simulink model "TTS_4motor_simplify_PMSM_ver2"  (R2020b)
settings: Solver=VariableStepAuto  StartTime=0.0  StopTime=0.8  RelTol=1e-3
InitFcn:
  | C = 0.015 % 中间直流电路的电容
  | f = 50 %频率
  | Rn = 0.01 % 整流部分电阻
  | Ln = 0.0012; % 整流电路部分电感
  | Udcref = 800*sqrt(2)
  | Un = 350
  | 
  | noiseDense = 1e-4 % 速度传感器故障噪声
  | 
  | w = 2*pi*f
  | 
  | np=2;
  | Tloadmax  = 50 % 最大负载
  | Tloadstart = 0.35 % 负载添加时间
  | Tdiscrete = 2e-6 % 离散时间
  | t_precharge = 0.15 % 整流预充电
  | Tpwm = 5e-4 % 逆变 PWM 周期
  | Ts = 1e-4
  | sample_time = Tdiscrete; % scope 采样时间
  | 
  | %基础参数
  | Rs_ref=0.43
  | Lm_ref=0.0006931
  | J_ref=0.1
  | Rflux_ref = 0.175
  | 
  | 
  | %电机 1 参数
  | Rflux1=0.9618*Rflux_ref
  | Rs1=0.9874*Rs_ref
  | Lm1=0.9747*Lm_ref
  | J1=0.9645*J_ref
  | 
  | 
  | %电机 2 参数
  | Rflux2=1.0145*Rflux_ref
  | Rs2=0.9810*Rs_ref
  | Lm2=0.9963*Lm_ref
  | J2=1.0415*J_ref
  | 
  | 
  | %电机 3 参数
  | Rflux3=1.0317*Rflux_ref
  | Rs3=0.9948*Rs_ref
  | Lm3=0.9914*Lm_ref
  | J3=1.0269*J_ref
  | 
  | 
  | %电机 4 参数
  | Rflux4=1.0481*Rflux_ref
  | Rs4=0.9914*Rs_ref
  | Lm4=0.9938*Lm_ref
  | J4=0.9873*J_ref
  | 
  | 
  | 
  | % 故障设置参数
  | % 速度传感器
  | tE1w = 10.3
  | 
  | % 逆变器
  | 
  | 
  | m1_pB = 0
  | m1_pC = 0
  | m1_t_inverter = 0.4 % 逆变器故障发生的时间
  | 
  | m2_pA = 0
  | m2_pB = 0
  | m2_pC = 0
  | m2_t_inverter = 0.4 % 逆变器故障发生的时间
  | 
  | m3_pA = 0
  | m3_pB = 0
  | m3_pC = 0
  | m3_t_inverter = 0.4 % 逆变器故障发生的时间
  | 
  | m4_pA = 0
  | m4_pB = 0
  | m4_pC = 0
  | m4_t_inverter = 0.4 % 逆变器故障发生的时间
undefined symbols (not defined in the file): m1_pA
libraries: powerlib x23, simulink x11, pid_lib x1, eeSinusoidalMeasurementV2 x1
(part 1 of 2)
settings Model: SimulationMode=accelerator  OrderedModelArguments=off  Creator=messer  LastModifiedBy=messer
settings SolverCC: ZeroCrossAlgorithm=Adaptive
settings DebuggingCC: IgnoredZcDiagnostic=none

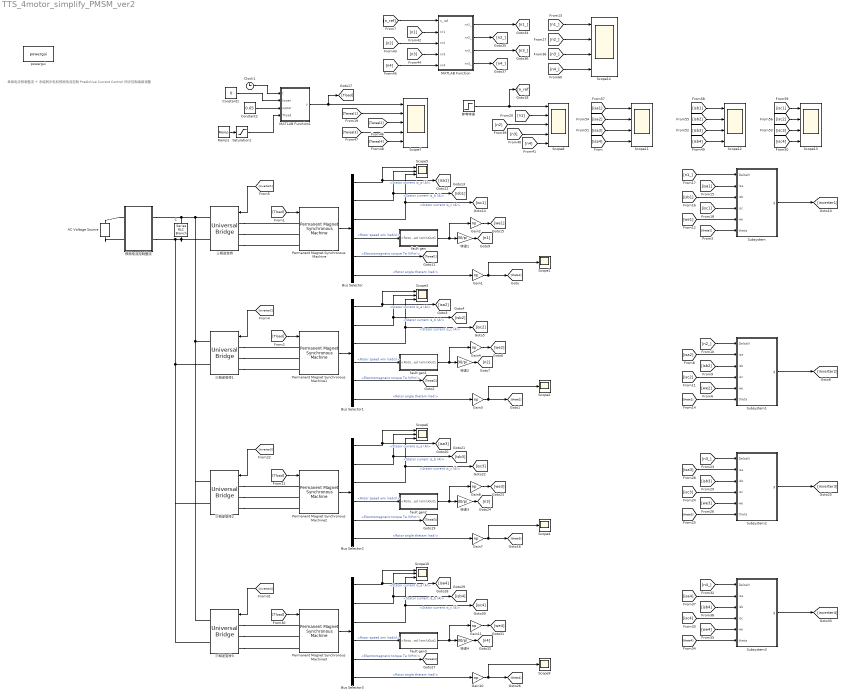
== system TTS_4motor_simplify_PMSM_ver2 ==
  note: 单相电流预测整流 + 永磁同步电机预测电流控制 Predictive Current Control
      |
      | 同步控制函数调整
  AC Voltage Source : powerlib/Electrical Sources/AC Voltage Source  Amplitude=Un  Phase=0  Frequency=50  SampleTime=0  Measurements=None  BusType=swing  Pref=10e3  Qref=0  Qmin=-inf  Qmax=+inf
  Bus Selector{,1..3} (4 alike) : BusSelector  OutputSignals=Stator current is_a (A),Stator current is_b (A),Stator current is_c (A),Rotor speed wm (rad/s),Electromagnetic torque Te (N*m),Rotor angle thetam (rad)
  C : powerlib/Elements/Series RLC Branch  LConnTagsString=__new0  RConnTagsString=__new0  BranchType=C  Resistance=0.05  Inductance=1e-3  SetiL0=off  InitialCurrent=0  Capacitance=C  Setx0=off  InitialVoltage=0  Measurements=None
  Clock1 : Clock
  Constant1 : Constant  Value=0
  Constant2 : Constant  Value=0.65
  Gain{1..4,7..8,10..11} (8 alike) : Gain  Gain=np
  MATLAB Function : MATLAB Function  TreatAsAtomicUnit=on
  MATLAB Function1 : MATLAB Function  TreatAsAtomicUnit=on
  Permanent Magnet Synchronous Machine : powerlib/Machines/Permanent Magnet Synchronous Machine  NbPhases=3  FluxDistribution=Sinusoidal  RotorType=Round  MechanicalLoad=Torque Tm  PresetModel=No  ShowDetailedParameters=on  MeasurementBus=off  Resistance=Rs1  Inductance=8.5e-3  dqInductances=[8.5e-3,8.5e-3]  La=Lm1  MachineConstant=Flux linkage established by magnets (V.s)  Flux=Rflux1  VoltageCst=63.483  TorqueCst=0.525  Flat=120  Mechanical=[J1 0.0 np 0]  PolePairs=4  InitialConditions=[0,0, 0,0]  InitialConditions5ph=[0 0 0 0 0 0]  RefAngle=Aligned with phase A axis (original Park)  IterativeDiscreteModel=Trapezoidal non iterative  TsBlock=-1  TsPowergui=0
  Permanent Magnet Synchronous Machine1 : powerlib/Machines/Permanent Magnet Synchronous Machine  NbPhases=3  FluxDistribution=Sinusoidal  RotorType=Round  MechanicalLoad=Torque Tm  PresetModel=No  ShowDetailedParameters=on  MeasurementBus=off  Resistance=Rs2  Inductance=8.5e-3  dqInductances=[8.5e-3,8.5e-3]  La=Lm2  MachineConstant=Flux linkage established by magnets (V.s)  Flux=Rflux2  VoltageCst=64.4035  TorqueCst=0.53261  Flat=120  Mechanical=[J2 0.0 np 0]  PolePairs=4  InitialConditions=[0,0, 0,0]  InitialConditions5ph=[0 0 0 0 0 0]  RefAngle=Aligned with phase A axis (original Park)  IterativeDiscreteModel=Trapezoidal non iterative  TsBlock=-1  TsPowergui=0
  Permanent Magnet Synchronous Machine2 : powerlib/Machines/Permanent Magnet Synchronous Machine  NbPhases=3  FluxDistribution=Sinusoidal  RotorType=Round  MechanicalLoad=Torque Tm  PresetModel=No  ShowDetailedParameters=on  MeasurementBus=off  Resistance=Rs3  Inductance=8.5e-3  dqInductances=[8.5e-3,8.5e-3]  La=Lm3  MachineConstant=Flux linkage established by magnets (V.s)  Flux=Rflux3  VoltageCst=65.4954  TorqueCst=0.54164  Flat=120  Mechanical=[J3 0.0 np 0]  PolePairs=4  InitialConditions=[0,0, 0,0]  InitialConditions5ph=[0 0 0 0 0 0]  RefAngle=Aligned with phase A axis (original Park)  IterativeDiscreteModel=Trapezoidal non iterative  TsBlock=-1  TsPowergui=0
  Permanent Magnet Synchronous Machine3 : powerlib/Machines/Permanent Magnet Synchronous Machine  NbPhases=3  FluxDistribution=Sinusoidal  RotorType=Round  MechanicalLoad=Torque Tm  PresetModel=No  ShowDetailedParameters=on  MeasurementBus=off  Resistance=Rs4  Inductance=8.5e-3  dqInductances=[8.5e-3,8.5e-3]  La=Lm4  MachineConstant=Flux linkage established by magnets (V.s)  Flux=Rflux4  VoltageCst=66.5365  TorqueCst=0.55025  Flat=120  Mechanical=[J4 0.0 np 0]  PolePairs=4  InitialConditions=[0,0, 0,0]  InitialConditions5ph=[0 0 0 0 0 0]  RefAngle=Aligned with phase A axis (original Park)  IterativeDiscreteModel=Trapezoidal non iterative  TsBlock=-1  TsPowergui=0
  Ramp1 : simulink/Sources/Ramp  slope=600  start=Tloadstart  InitialOutput=0
  Saturation1 : Saturate  UpperLimit=Tloadmax  LowerLimit=0
  Scope{1..2,4,9} (4 alike) : Scope
  Scope{3,5..6,10} (4 alike) : Scope  NumInputPorts=3
  Scope{11..14} (4 alike) : Scope  NumInputPorts=4
  Scope7 : Scope  NumInputPorts=5
  Scope8 : Scope  NumInputPorts=5
  Subsystem : Subsystem
  Subsystem1 : Subsystem
  Subsystem2 : Subsystem
  Subsystem3 : Subsystem
  fault gen : Subsystem
  fault gen1 : Subsystem
  fault gen2 : Subsystem
  fault gen3 : Subsystem
  powergui : powerlib/powergui  Priority=1  SimulationMode=Discrete  SampleTime=1e-6  frequency=60  Iterations=50  frequencyindice=0  Pbase=100e6  ErrMax=1e-4  UnitsV=kV  UnitsW=MW  buscounter=0  FunctionMessages=off  echomessages=off  EnableUseOfTLC=off  CurrentSourceSwitches=off  DisableSnubberDevices=off  DisableRonSwitches=off  DisableVfSwitches=off  DisplayEquations=off  AutomaticDiscreteSolvers=off  SolverType=Tustin/Backward Euler (TBE)  Interpol=off  ExternalGateDelay=off  methode=off  Ts=100  x0status=blocks  SPID=on  SwTol=0  HookPort=off  NonlinearTolerance=1e-4  nMaxIteration=100  ContinueOnMaxIteration=off  RestoreLinks=warning  ResistiveCurrentMeasurement=off  Frange=[0:2:500]  Ylog=off  Xlog=on  ShowGrid=off  save=off  variable=ZData  structure=0  ZoomFFT=off  StartTime=0.0  cycles=1  DisplayStyle=1  fundamental=60  FreqAxis=off  MaxFrequency=1000  frequencyindicesteady=1  RmsSteady=1  display=off
  三相逆变桥{,1..3} (4 alike) : powerlib/Power Electronics/Universal Bridge  Arms=3  SnubberResistance=1e5  SnubberCapacitance=inf  Device=IGBT / Diodes  Ron=1e-3  Lon=0  ForwardVoltages="[  0  0  ]"  ForwardVoltage=0  GTOparameters=[ 10e-6 , 20e-6 ]  IGBTparameters=[ 1e-6 , 2e-6 ]  Measurements=None  Measurements_2=None  converterType=Rectifier
  参考转速 : Step  Time=0.05  After=1800  SampleTime=0
  转速{1..4} (4 alike) : Gain  Gain=30/pi
  预测电流控制整流 : Subsystem
  wires:
  Bus Selector/5 -> [Tereal1]  "<Electromagnetic torque Te (N*m)>"
  转速1/1 -> [n1]
  Bus Selector/2 -> Scope5/2, [isb1]  "<Stator current is_b (A)>"
  fault gen/1(Out1) -> Gain2/1, 转速1/1
  Gain2/1 -> [we1]
  Bus Selector/4 -> fault gen/1(<Rotor speed (wm)>)  "<Rotor speed wm (rad/s)>"
  Bus Selector/3 -> [isc1], Scope5/3  "<Stator current is_c (A)>"
  Bus Selector/1 -> Scope5/1, [isa1]  "<Stator current is_a (A)>"
  Permanent Magnet Synchronous Machine/1 -> Bus Selector/1
  [isb1] -> Subsystem/3(isb)
  [we1] -> Subsystem/5(we)
  Subsystem/1(g) -> [inverter1]
  [isc1] -> Subsystem/4(isc)
  [n1_] -> Subsystem/1(DeltaN)
  [isa1] -> Subsystem/2(isa)
  Saturation1/1 -> MATLAB Function1/4(Tload)
  Constant1/1 -> MATLAB Function1/2(lower)
  Constant2/1 -> MATLAB Function1/3(upper)
  MATLAB Function1/1(y) -> Scope7/1, [Tload]
  [Tereal1] -> Scope7/2
  Clock1/1 -> MATLAB Function1/1(t)
  Ramp1/1 -> Saturation1/1
  [n1] -> Scope8/2
  Bus Selector/6 -> Gain1/1  "<Rotor angle thetam (rad)>"
  [inverter1] -> 三相逆变桥/1
  [theta1] -> Subsystem/6(theta)
  Gain1/1 -> Scope1/1, [theta1]
  [Tload] -> Permanent Magnet Synchronous Machine/1
  参考转速/1 -> Scope8/1, [n_ref]
  [Tload] -> Permanent Magnet Synchronous Machine1/1
  Gain3/1 -> [theta2], Scope2/1
  [inverter2] -> 三相逆变桥1/1
  Bus Selector1/6 -> Gain3/1  "<Rotor angle thetam (rad)>"
  Permanent Magnet Synchronous Machine1/1 -> Bus Selector1/1
  Bus Selector1/1 -> [isa2], Scope3/1  "<Stator current is_a (A)>"
  Bus Selector1/3 -> Scope3/3, [isc2]  "<Stator current is_c (A)>"
  Bus Selector1/4 -> fault gen1/1(<Rotor speed (wm)>)  "<Rotor speed wm (rad/s)>"
  Gain4/1 -> [we2]
  fault gen1/1(Out1) -> 转速2/1, Gain4/1
  Bus Selector1/2 -> [isb2], Scope3/2  "<Stator current is_b (A)>"
  转速2/1 -> [n2]
  Bus Selector1/5 -> [Tereal2]  "<Electromagnetic torque Te (N*m)>"
  [theta2] -> Subsystem1/6(theta)
  [isa2] -> Subsystem1/2(isa)
  [isc2] -> Subsystem1/4(isc)
  Subsystem1/1(g) -> [inverter2]
  [we2] -> Subsystem1/5(we)
  [isb2] -> Subsystem1/3(isb)
  [n2_] -> Subsystem1/1(DeltaN)
  Bus Selector2/5 -> [Tereal3]  "<Electromagnetic torque Te (N*m)>"
  转速3/1 -> [n3]
  Bus Selector2/2 -> Scope6/2, [isb3]  "<Stator current is_b (A)>"
  fault gen2/1(Out1) -> Gain8/1, 转速3/1
  Gain8/1 -> [we3]
  Bus Selector2/4 -> fault gen2/1(<Rotor speed (wm)>)  "<Rotor speed wm (rad/s)>"
  Bus Selector2/3 -> [isc3], Scope6/3  "<Stator current is_c (A)>"
  Bus Selector2/1 -> Scope6/1, [isa3]  "<Stator current is_a (A)>"
  Permanent Magnet Synchronous Machine2/1 -> Bus Selector2/1
  Bus Selector2/6 -> Gain7/1  "<Rotor angle thetam (rad)>"
  [inverter3] -> 三相逆变桥2/1
  Gain7/1 -> Scope4/1, [theta3]
  [Tload] -> Permanent Magnet Synchronous Machine2/1
  [n3_] -> Subsystem2/1(DeltaN)
  [isb3] -> Subsystem2/3(isb)
  [we3] -> Subsystem2/5(we)
  Subsystem2/1(g) -> [inverter3]
  [isc3] -> Subsystem2/4(isc)
  [isa3] -> Subsystem2/2(isa)
  [theta3] -> Subsystem2/6(theta)
  [Tload] -> Permanent Magnet Synchronous Machine3/1
  Gain10/1 -> [theta4], Scope9/1
  [inverter4] -> 三相逆变桥3/1
  Bus Selector3/6 -> Gain10/1  "<Rotor angle thetam (rad)>"
  Permanent Magnet Synchronous Machine3/1 -> Bus Selector3/1
  Bus Selector3/1 -> [isa4], Scope10/1  "<Stator current is_a (A)>"
  Bus Selector3/3 -> Scope10/3, [isc4]  "<Stator current is_c (A)>"
  Bus Selector3/4 -> fault gen3/1(<Rotor speed (wm)>)  "<Rotor speed wm (rad/s)>"
  Gain11/1 -> [we4]
  fault gen3/1(Out1) -> 转速4/1, Gain11/1
  Bus Selector3/2 -> [isb4], Scope10/2  "<Stator current is_b (A)>"
  转速4/1 -> [n4]
  Bus Selector3/5 -> [Tereal4]  "<Electromagnetic torque Te (N*m)>"
  [theta4] -> Subsystem3/6(theta)
  [isa4] -> Subsystem3/2(isa)
  [isc4] -> Subsystem3/4(isc)
  Subsystem3/1(g) -> [inverter4]
  [we4] -> Subsystem3/5(we)
  [isb4] -> Subsystem3/3(isb)
  [n4_] -> Subsystem3/1(DeltaN)
  [n2] -> Scope8/3
  [n3] -> Scope8/4
  [n4] -> Scope8/5
  [n1] -> MATLAB Function/2(nr1)
  [n2] -> MATLAB Function/3(nr2)
  [n3] -> MATLAB Function/4(nr3)
  [n4] -> MATLAB Function/5(nr4)
  MATLAB Function/1(nr1_) -> [n1_]
  MATLAB Function/4(nr4_) -> [n4_]
  MATLAB Function/3(nr3_) -> [n3_]
  MATLAB Function/2(nr2_) -> [n2_]
  [Tereal2] -> Scope7/3
  [Tereal3] -> Scope7/4
  [Tereal4] -> Scope7/5
  [isa1] -> Scope11/1
  [isa2] -> Scope11/2
  [isa3] -> Scope11/3
  [isa4] -> Scope11/4
  [isb1] -> Scope12/1
  [isb2] -> Scope12/2
  [isb3] -> Scope12/3
  [isb4] -> Scope12/4
  [isc1] -> Scope13/1
  [isc2] -> Scope13/2
  [isc3] -> Scope13/3
  [isc4] -> Scope13/4
  [n_ref] -> MATLAB Function/1(n_ref)
  [n1_] -> Scope14/1
  [n2_] -> Scope14/2
  [n3_] -> Scope14/3
  [n4_] -> Scope14/4
  connections:
  预测电流控制整流/RConn2 -- 三相逆变桥3/RConn2 -- 三相逆变桥2/RConn2 -- 三相逆变桥1/RConn2 -- C/RConn1 -- 三相逆变桥/RConn2
  预测电流控制整流/RConn1 -- C/LConn1 -- 三相逆变桥3/RConn1 -- 三相逆变桥2/RConn1 -- 三相逆变桥1/RConn1 -- 三相逆变桥/RConn1
  三相逆变桥/LConn1 -- Permanent Magnet Synchronous Machine/LConn1
  三相逆变桥/LConn2 -- Permanent Magnet Synchronous Machine/LConn2
  三相逆变桥/LConn3 -- Permanent Magnet Synchronous Machine/LConn3
  AC Voltage Source/LConn1 -- 预测电流控制整流/LConn2
  预测电流控制整流/LConn1 -- AC Voltage Source/RConn1
  三相逆变桥1/LConn1 -- Permanent Magnet Synchronous Machine1/LConn1
  三相逆变桥1/LConn2 -- Permanent Magnet Synchronous Machine1/LConn2
  三相逆变桥1/LConn3 -- Permanent Magnet Synchronous Machine1/LConn3
  三相逆变桥2/LConn2 -- Permanent Magnet Synchronous Machine2/LConn2
  三相逆变桥2/LConn1 -- Permanent Magnet Synchronous Machine2/LConn1
  三相逆变桥2/LConn3 -- Permanent Magnet Synchronous Machine2/LConn3
  三相逆变桥3/LConn1 -- Permanent Magnet Synchronous Machine3/LConn1
  三相逆变桥3/LConn2 -- Permanent Magnet Synchronous Machine3/LConn2
  三相逆变桥3/LConn3 -- Permanent Magnet Synchronous Machine3/LConn3

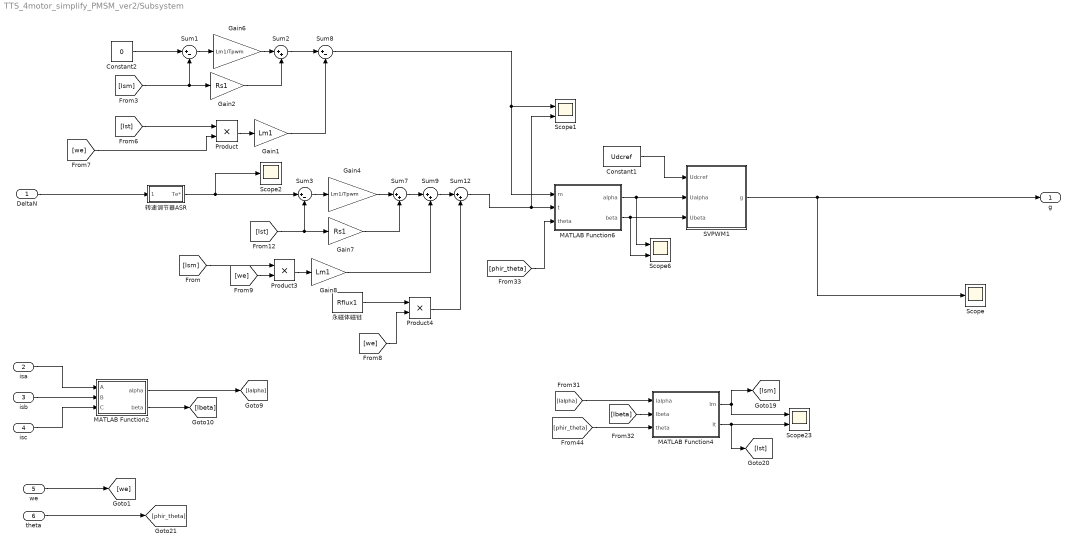
== system TTS_4motor_simplify_PMSM_ver2/Subsystem ==
  DeltaN : Inport
  isa : Inport  Port=2
  isb : Inport  Port=3
  isc : Inport  Port=4
  we : Inport  Port=5
  theta : Inport  Port=6
  Constant1 : Constant  Value=Udcref
  Constant2 : Constant  Value=0
  Gain1 : Gain  Gain=Lm1
  Gain2 : Gain  Gain=Rs1
  Gain4 : Gain  Gain=Lm1/Tpwm
  Gain6 : Gain  Gain=Lm1/Tpwm
  Gain7 : Gain  Gain=Rs1
  Gain8 : Gain  Gain=Lm1
  MATLAB Function2 : MATLAB Function  TreatAsAtomicUnit=on
  MATLAB Function4 : MATLAB Function  TreatAsAtomicUnit=on
  MATLAB Function6 : MATLAB Function  TreatAsAtomicUnit=on
  Product : Product
  Product3 : Product
  Product4 : Product
  SVPWM1 : Subsystem
  Scope : Scope
  Scope1 : Scope  NumInputPorts=2
  Scope2 : Scope
  Scope23 : Scope  NumInputPorts=2
  Scope6 : Scope  NumInputPorts=2
  Sum1 : Sum  Inputs=|+-
  Sum{2,7,9,12} (4 alike) : Sum  Inputs=|++
  Sum3 : Sum  Inputs=|+-
  Sum8 : Sum  Inputs=|+-
  永磁体磁链 : Constant  Value=Rflux1
  转速调节器ASR : Subsystem
  g : Outport
  wires:
  Constant1/1 -> SVPWM1/1(Udcref)
  MATLAB Function4/1(Im) -> [Ism], Scope23/1
  isc/1 -> MATLAB Function2/3(C)
  we/1 -> [we]
  MATLAB Function6/1(alpha) -> SVPWM1/2(Ualpha), Scope6/1
  [phir_theta] -> MATLAB Function6/3(theta)
  MATLAB Function4/2(It) -> Scope23/2, [Ist]
  isb/1 -> MATLAB Function2/2(B)
  MATLAB Function6/2(beta) -> Scope6/2, SVPWM1/3(Ubeta)
  [phir_theta] -> MATLAB Function4/3(theta)
  DeltaN/1 -> 转速调节器ASR/1("  ")
  SVPWM1/1(g) -> Scope/1, g/1
  MATLAB Function2/2(beta) -> [Ibeta]
  [Ibeta] -> MATLAB Function4/2(Ibeta)
  MATLAB Function2/1(alpha) -> [Ialpha]
  [Ialpha] -> MATLAB Function4/1(Ialpha)
  isa/1 -> MATLAB Function2/1(A)
  [Ist] -> Product/1
  [we] -> Product/2
  [Ism] -> Gain2/1, Sum1/2
  Sum1/1 -> Gain6/1
  [Ism] -> Product3/1
  [we] -> Product3/2
  转速调节器ASR/1(Te*) -> Scope2/1, Sum3/1
  Sum3/1 -> Gain4/1
  Sum7/1 -> Sum9/1
  Gain6/1 -> Sum2/1
  Gain2/1 -> Sum2/2
  Sum2/1 -> Sum8/1
  Product/1 -> Gain1/1
  Gain1/1 -> Sum8/2
  [Ist] -> Gain7/1, Sum3/2
  Gain4/1 -> Sum7/1
  Gain7/1 -> Sum7/2
  Product3/1 -> Gain8/1
  Sum9/1 -> Sum12/1
  Gain8/1 -> Sum9/2
  [we] -> Product4/2
  永磁体磁链/1 -> Product4/1
  Product4/1 -> Sum12/2
  Constant2/1 -> Sum1/1
  Sum8/1 -> MATLAB Function6/1(m), Scope1/1
  Sum12/1 -> MATLAB Function6/2(t), Scope1/2
  theta/1 -> [phir_theta]

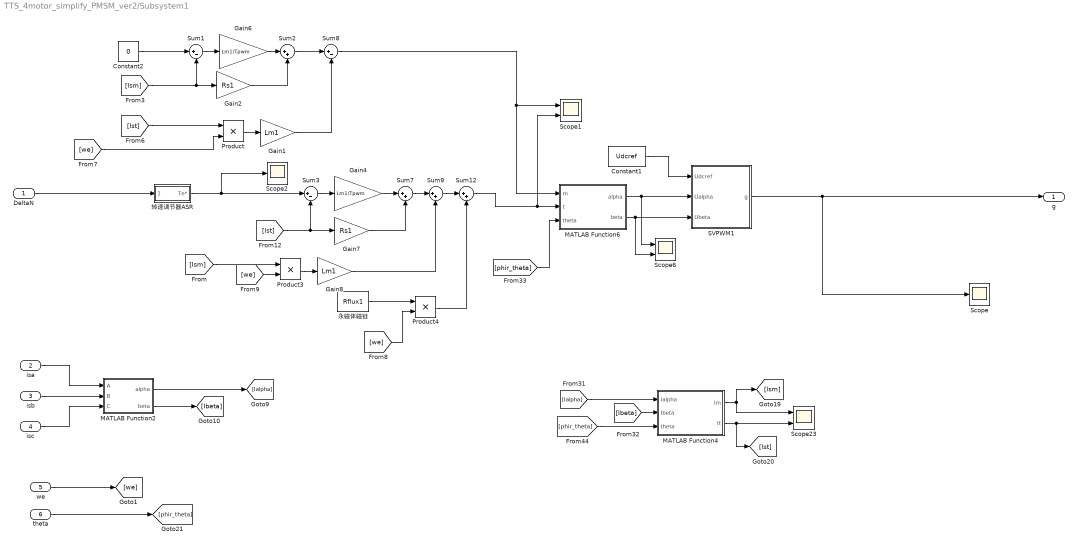
== system TTS_4motor_simplify_PMSM_ver2/Subsystem1 ==
  DeltaN : Inport
  isa : Inport  Port=2
  isb : Inport  Port=3
  isc : Inport  Port=4
  we : Inport  Port=5
  theta : Inport  Port=6
  Constant1 : Constant  Value=Udcref
  Constant2 : Constant  Value=0
  Gain1 : Gain  Gain=Lm1
  Gain2 : Gain  Gain=Rs1
  Gain4 : Gain  Gain=Lm1/Tpwm
  Gain6 : Gain  Gain=Lm1/Tpwm
  Gain7 : Gain  Gain=Rs1
  Gain8 : Gain  Gain=Lm1
  MATLAB Function2 : MATLAB Function  TreatAsAtomicUnit=on
  MATLAB Function4 : MATLAB Function  TreatAsAtomicUnit=on
  MATLAB Function6 : MATLAB Function  TreatAsAtomicUnit=on
  Product : Product
  Product3 : Product
  Product4 : Product
  SVPWM1 : Subsystem
  Scope : Scope
  Scope1 : Scope  NumInputPorts=2
  Scope2 : Scope
  Scope23 : Scope  NumInputPorts=2
  Scope6 : Scope  NumInputPorts=2
  Sum1 : Sum  Inputs=|+-
  Sum{2,7,9,12} (4 alike) : Sum  Inputs=|++
  Sum3 : Sum  Inputs=|+-
  Sum8 : Sum  Inputs=|+-
  永磁体磁链 : Constant  Value=Rflux1
  转速调节器ASR : Subsystem
  g : Outport
  wires:
  theta/1 -> [phir_theta]
  Sum12/1 -> Scope1/2, MATLAB Function6/2(t)
  Sum8/1 -> Scope1/1, MATLAB Function6/1(m)
  Constant2/1 -> Sum1/1
  Product4/1 -> Sum12/2
  永磁体磁链/1 -> Product4/1
  [we] -> Product4/2
  Gain8/1 -> Sum9/2
  Sum9/1 -> Sum12/1
  Product3/1 -> Gain8/1
  Gain7/1 -> Sum7/2
  Gain4/1 -> Sum7/1
  [Ist] -> Sum3/2, Gain7/1
  Gain1/1 -> Sum8/2
  Product/1 -> Gain1/1
  Sum2/1 -> Sum8/1
  Gain2/1 -> Sum2/2
  Gain6/1 -> Sum2/1
  Sum7/1 -> Sum9/1
  Sum3/1 -> Gain4/1
  转速调节器ASR/1(Te*) -> Sum3/1, Scope2/1
  [we] -> Product3/2
  [Ism] -> Product3/1
  Sum1/1 -> Gain6/1
  [Ism] -> Sum1/2, Gain2/1
  [we] -> Product/2
  [Ist] -> Product/1
  isa/1 -> MATLAB Function2/1(A)
  [Ialpha] -> MATLAB Function4/1(Ialpha)
  MATLAB Function2/1(alpha) -> [Ialpha]
  [Ibeta] -> MATLAB Function4/2(Ibeta)
  MATLAB Function2/2(beta) -> [Ibeta]
  SVPWM1/1(g) -> g/1, Scope/1
  DeltaN/1 -> 转速调节器ASR/1("  ")
  [phir_theta] -> MATLAB Function4/3(theta)
  MATLAB Function6/2(beta) -> SVPWM1/3(Ubeta), Scope6/2
  isb/1 -> MATLAB Function2/2(B)
  MATLAB Function4/2(It) -> [Ist], Scope23/2
  [phir_theta] -> MATLAB Function6/3(theta)
  MATLAB Function6/1(alpha) -> Scope6/1, SVPWM1/2(Ualpha)
  we/1 -> [we]
  isc/1 -> MATLAB Function2/3(C)
  MATLAB Function4/1(Im) -> Scope23/1, [Ism]
  Constant1/1 -> SVPWM1/1(Udcref)

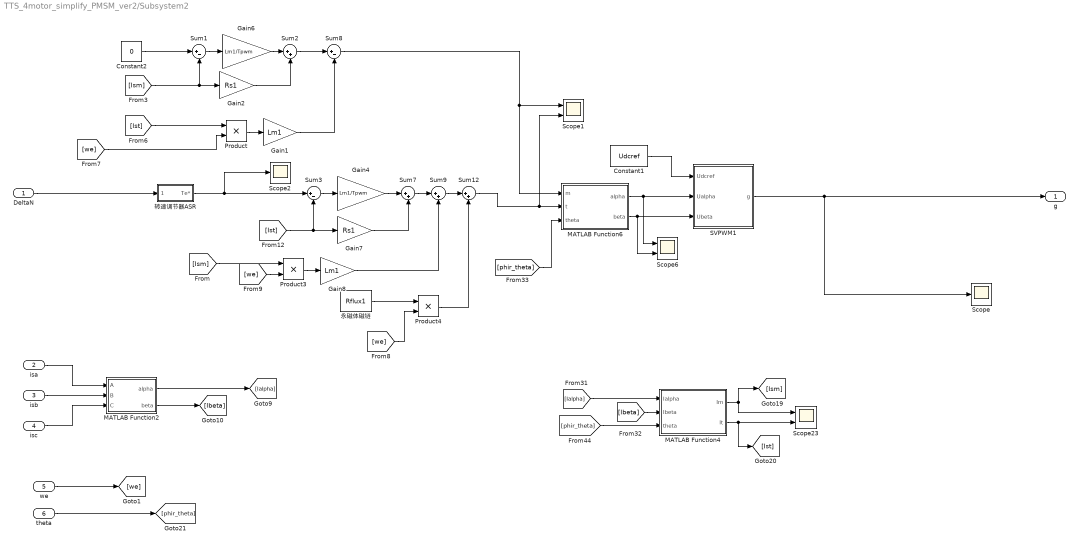
== system TTS_4motor_simplify_PMSM_ver2/Subsystem2 ==
  DeltaN : Inport
  isa : Inport  Port=2
  isb : Inport  Port=3
  isc : Inport  Port=4
  we : Inport  Port=5
  theta : Inport  Port=6
  Constant1 : Constant  Value=Udcref
  Constant2 : Constant  Value=0
  Gain1 : Gain  Gain=Lm1
  Gain2 : Gain  Gain=Rs1
  Gain4 : Gain  Gain=Lm1/Tpwm
  Gain6 : Gain  Gain=Lm1/Tpwm
  Gain7 : Gain  Gain=Rs1
  Gain8 : Gain  Gain=Lm1
  MATLAB Function2 : MATLAB Function  TreatAsAtomicUnit=on
  MATLAB Function4 : MATLAB Function  TreatAsAtomicUnit=on
  MATLAB Function6 : MATLAB Function  TreatAsAtomicUnit=on
  Product : Product
  Product3 : Product
  Product4 : Product
  SVPWM1 : Subsystem
  Scope : Scope
  Scope1 : Scope  NumInputPorts=2
  Scope2 : Scope
  Scope23 : Scope  NumInputPorts=2
  Scope6 : Scope  NumInputPorts=2
  Sum1 : Sum  Inputs=|+-
  Sum{2,7,9,12} (4 alike) : Sum  Inputs=|++
  Sum3 : Sum  Inputs=|+-
  Sum8 : Sum  Inputs=|+-
  永磁体磁链 : Constant  Value=Rflux1
  转速调节器ASR : Subsystem
  g : Outport
  wires:
  Constant1/1 -> SVPWM1/1(Udcref)
  MATLAB Function4/1(Im) -> [Ism], Scope23/1
  isc/1 -> MATLAB Function2/3(C)
  we/1 -> [we]
  MATLAB Function6/1(alpha) -> SVPWM1/2(Ualpha), Scope6/1
  [phir_theta] -> MATLAB Function6/3(theta)
  MATLAB Function4/2(It) -> Scope23/2, [Ist]
  isb/1 -> MATLAB Function2/2(B)
  MATLAB Function6/2(beta) -> Scope6/2, SVPWM1/3(Ubeta)
  [phir_theta] -> MATLAB Function4/3(theta)
  DeltaN/1 -> 转速调节器ASR/1("  ")
  SVPWM1/1(g) -> Scope/1, g/1
  MATLAB Function2/2(beta) -> [Ibeta]
  [Ibeta] -> MATLAB Function4/2(Ibeta)
  MATLAB Function2/1(alpha) -> [Ialpha]
  [Ialpha] -> MATLAB Function4/1(Ialpha)
  isa/1 -> MATLAB Function2/1(A)
  [Ist] -> Product/1
  [we] -> Product/2
  [Ism] -> Gain2/1, Sum1/2
  Sum1/1 -> Gain6/1
  [Ism] -> Product3/1
  [we] -> Product3/2
  转速调节器ASR/1(Te*) -> Scope2/1, Sum3/1
  Sum3/1 -> Gain4/1
  Sum7/1 -> Sum9/1
  Gain6/1 -> Sum2/1
  Gain2/1 -> Sum2/2
  Sum2/1 -> Sum8/1
  Product/1 -> Gain1/1
  Gain1/1 -> Sum8/2
  [Ist] -> Gain7/1, Sum3/2
  Gain4/1 -> Sum7/1
  Gain7/1 -> Sum7/2
  Product3/1 -> Gain8/1
  Sum9/1 -> Sum12/1
  Gain8/1 -> Sum9/2
  [we] -> Product4/2
  永磁体磁链/1 -> Product4/1
  Product4/1 -> Sum12/2
  Constant2/1 -> Sum1/1
  Sum8/1 -> MATLAB Function6/1(m), Scope1/1
  Sum12/1 -> MATLAB Function6/2(t), Scope1/2
  theta/1 -> [phir_theta]

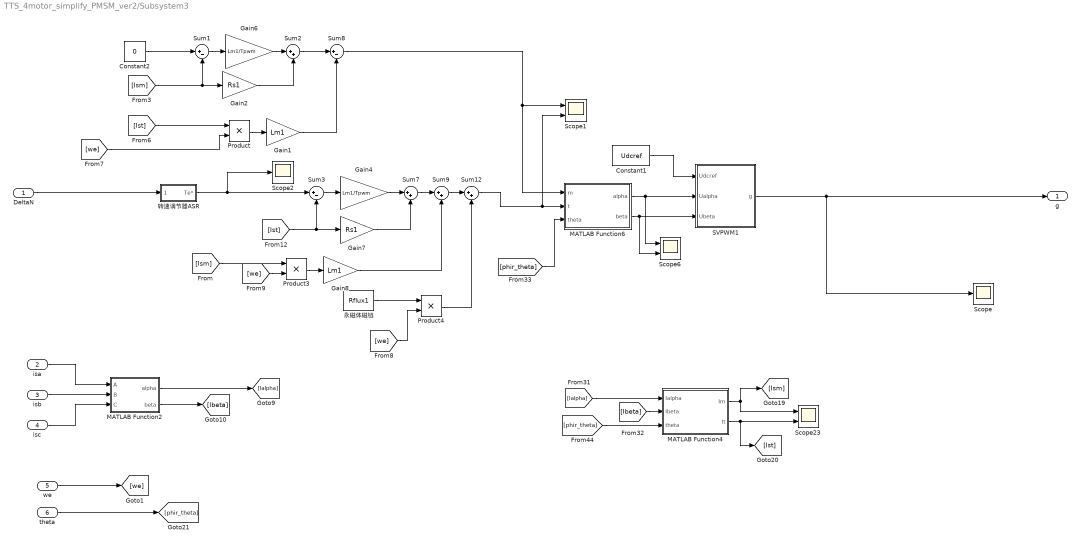
== system TTS_4motor_simplify_PMSM_ver2/Subsystem3 ==
  DeltaN : Inport
  isa : Inport  Port=2
  isb : Inport  Port=3
  isc : Inport  Port=4
  we : Inport  Port=5
  theta : Inport  Port=6
  Constant1 : Constant  Value=Udcref
  Constant2 : Constant  Value=0
  Gain1 : Gain  Gain=Lm1
  Gain2 : Gain  Gain=Rs1
  Gain4 : Gain  Gain=Lm1/Tpwm
  Gain6 : Gain  Gain=Lm1/Tpwm
  Gain7 : Gain  Gain=Rs1
  Gain8 : Gain  Gain=Lm1
  MATLAB Function2 : MATLAB Function  TreatAsAtomicUnit=on
  MATLAB Function4 : MATLAB Function  TreatAsAtomicUnit=on
  MATLAB Function6 : MATLAB Function  TreatAsAtomicUnit=on
  Product : Product
  Product3 : Product
  Product4 : Product
  SVPWM1 : Subsystem
  Scope : Scope
  Scope1 : Scope  NumInputPorts=2
  Scope2 : Scope
  Scope23 : Scope  NumInputPorts=2
  Scope6 : Scope  NumInputPorts=2
  Sum1 : Sum  Inputs=|+-
  Sum{2,7,9,12} (4 alike) : Sum  Inputs=|++
  Sum3 : Sum  Inputs=|+-
  Sum8 : Sum  Inputs=|+-
  永磁体磁链 : Constant  Value=Rflux1
  转速调节器ASR : Subsystem
  g : Outport
  wires:
  theta/1 -> [phir_theta]
  Sum12/1 -> Scope1/2, MATLAB Function6/2(t)
  Sum8/1 -> Scope1/1, MATLAB Function6/1(m)
  Constant2/1 -> Sum1/1
  Product4/1 -> Sum12/2
  永磁体磁链/1 -> Product4/1
  [we] -> Product4/2
  Gain8/1 -> Sum9/2
  Sum9/1 -> Sum12/1
  Product3/1 -> Gain8/1
  Gain7/1 -> Sum7/2
  Gain4/1 -> Sum7/1
  [Ist] -> Sum3/2, Gain7/1
  Gain1/1 -> Sum8/2
  Product/1 -> Gain1/1
  Sum2/1 -> Sum8/1
  Gain2/1 -> Sum2/2
  Gain6/1 -> Sum2/1
  Sum7/1 -> Sum9/1
  Sum3/1 -> Gain4/1
  转速调节器ASR/1(Te*) -> Sum3/1, Scope2/1
  [we] -> Product3/2
  [Ism] -> Product3/1
  Sum1/1 -> Gain6/1
  [Ism] -> Sum1/2, Gain2/1
  [we] -> Product/2
  [Ist] -> Product/1
  isa/1 -> MATLAB Function2/1(A)
  [Ialpha] -> MATLAB Function4/1(Ialpha)
  MATLAB Function2/1(alpha) -> [Ialpha]
  [Ibeta] -> MATLAB Function4/2(Ibeta)
  MATLAB Function2/2(beta) -> [Ibeta]
  SVPWM1/1(g) -> g/1, Scope/1
  DeltaN/1 -> 转速调节器ASR/1("  ")
  [phir_theta] -> MATLAB Function4/3(theta)
  MATLAB Function6/2(beta) -> SVPWM1/3(Ubeta), Scope6/2
  isb/1 -> MATLAB Function2/2(B)
  MATLAB Function4/2(It) -> [Ist], Scope23/2
  [phir_theta] -> MATLAB Function6/3(theta)
  MATLAB Function6/1(alpha) -> Scope6/1, SVPWM1/2(Ualpha)
  we/1 -> [we]
  isc/1 -> MATLAB Function2/3(C)
  MATLAB Function4/1(Im) -> Scope23/1, [Ism]
  Constant1/1 -> SVPWM1/1(Udcref)

== system TTS_4motor_simplify_PMSM_ver2/fault gen ==
  <Rotor speed (wm)> : Inport
  Band-Limited White Noise1 : simulink/Sources/Band-Limited White Noise  Cov=[0.08]  Ts=noiseDense  seed=[23341]
  Clock : Clock
  Gain : Gain
  Sum2 : Sum  Inputs=++|
  Switch : Switch  Criteria=u2 > Threshold  Threshold=tE1w
  Out1 : Outport
  wires:
  Clock/1 -> Switch/2
  Switch/1 -> Out1/1
  Sum2/1 -> Switch/1
  <Rotor speed (wm)>/1 -> Switch/3, Gain/1
  Band-Limited White Noise1/1 -> Sum2/1
  Gain/1 -> Sum2/2

== system TTS_4motor_simplify_PMSM_ver2/fault gen1 ==
  <Rotor speed (wm)> : Inport
  Band-Limited White Noise1 : simulink/Sources/Band-Limited White Noise  Cov=[0.08]  Ts=noiseDense  seed=[23341]
  Clock : Clock
  Gain : Gain
  Sum2 : Sum  Inputs=++|
  Switch : Switch  Criteria=u2 > Threshold  Threshold=tE1w
  Out1 : Outport
  wires:
  Gain/1 -> Sum2/2
  Band-Limited White Noise1/1 -> Sum2/1
  <Rotor speed (wm)>/1 -> Gain/1, Switch/3
  Sum2/1 -> Switch/1
  Switch/1 -> Out1/1
  Clock/1 -> Switch/2

== system TTS_4motor_simplify_PMSM_ver2/fault gen2 ==
  <Rotor speed (wm)> : Inport
  Band-Limited White Noise1 : simulink/Sources/Band-Limited White Noise  Cov=[0.08]  Ts=noiseDense  seed=[23341]
  Clock : Clock
  Gain : Gain
  Sum2 : Sum  Inputs=++|
  Switch : Switch  Criteria=u2 > Threshold  Threshold=tE1w
  Out1 : Outport
  wires:
  Clock/1 -> Switch/2
  Switch/1 -> Out1/1
  Sum2/1 -> Switch/1
  <Rotor speed (wm)>/1 -> Switch/3, Gain/1
  Band-Limited White Noise1/1 -> Sum2/1
  Gain/1 -> Sum2/2

== system TTS_4motor_simplify_PMSM_ver2/fault gen3 ==
  <Rotor speed (wm)> : Inport
  Band-Limited White Noise1 : simulink/Sources/Band-Limited White Noise  Cov=[0.08]  Ts=noiseDense  seed=[23341]
  Clock : Clock
  Gain : Gain
  Sum2 : Sum  Inputs=++|
  Switch : Switch  Criteria=u2 > Threshold  Threshold=tE1w
  Out1 : Outport
  wires:
  Gain/1 -> Sum2/2
  Band-Limited White Noise1/1 -> Sum2/1
  <Rotor speed (wm)>/1 -> Gain/1, Switch/3
  Sum2/1 -> Switch/1
  Switch/1 -> Out1/1
  Clock/1 -> Switch/2

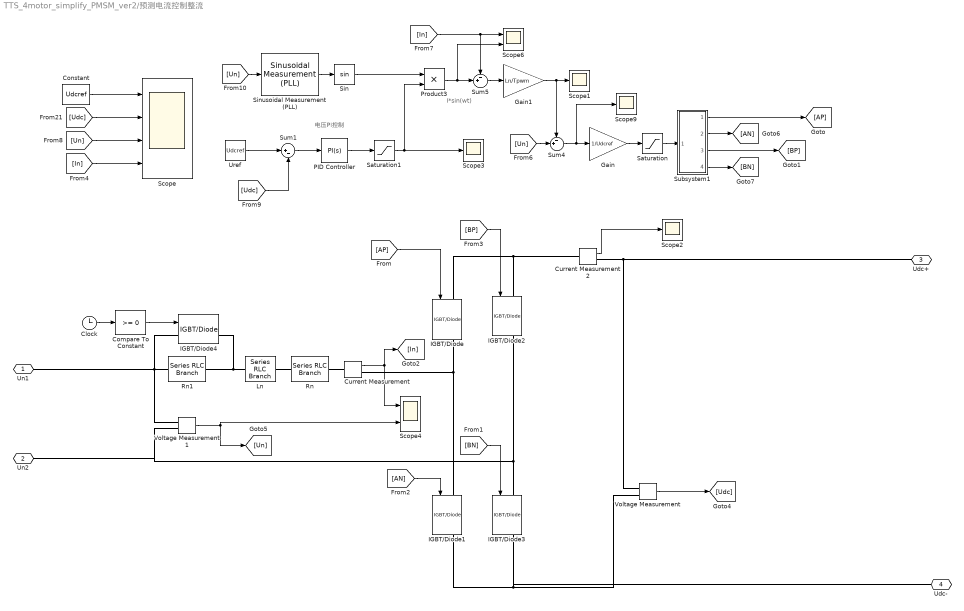
== system TTS_4motor_simplify_PMSM_ver2/预测电流控制整流 ==
  note: 电压PI控制
  note: I*sin(wt)
  Clock : Clock
  Compare To Constant : simulink/Logic and Bit Operations/Compare To Constant  relop=>=  const=0  OutDataTypeStr=boolean
  Constant : Constant  Value=Udcref
  Current Measurement : powerlib/Measurements/Current Measurement  PhasorSimulation=off  OutputType=Complex  PSBequivalent=0
  Current Measurement2 : powerlib/Measurements/Current Measurement  PhasorSimulation=off  OutputType=Complex  PSBequivalent=0
  Gain : Gain  Gain=1/Udcref
  Gain1 : Gain  Gain=Ln/Tpwm
  IGBT/Diode{,1..4} (5 alike) : powerlib/Power Electronics/IGBT//Diode  Ron=1e-3  Rs=1e5  Cs=inf  Measurements=on
  Ln : powerlib/Elements/Series RLC Branch  LConnTagsString=__new0  RConnTagsString=__new0  BranchType=L  Resistance=1  Inductance=Ln  SetiL0=off  InitialCurrent=0  Capacitance=1e-6  Setx0=off  InitialVoltage=0  Measurements=None
  PID Controller : pid_lib/PID Controller  Controller=PI  Form=Parallel  TimeDomain=Continuous-time  UseExternalTs=off  SampleTime=-1  IntegratorMethod=Forward Euler  FilterMethod=Forward Euler  ControllerParametersSource=internal  P=7  I=3  D=0  UseFilter=on  N=100  TunerSelectOption=Transfer Function Based (PID Tuner App)  InitialConditionSource=internal  InitialConditionForIntegrator=0  InitialConditionForFilter=0  DifferentiatorICPrevScaledInput=0  ExternalReset=none  TrackingMode=off  Kt=1  LimitOutput=off  SatLimitsSource=internal  UpperSaturationLimit=inf  LowerSaturationLimit=-inf  LinearizeAsGain=on  AntiWindupMode=none  Kb=1  POutMin=[]  POutMax=[]  IOutMin=[]  IOutMax=[]  DOutMin=[]  DOutMax=[]  NOutMin=[]  NOutMax=[]  SumOutMin=[]  SumOutMax=[]  SaturationOutMin=[]  SaturationOutMax=[]  PParamMin=[]  PParamMax=[]  IParamMin=[]  IParamMax=[]  DParamMin=[]  DParamMax=[]  NParamMin=[]  NParamMax=[]  KbParamMin=[]  KbParamMax=[]  KtParamMin=[]  KtParamMax=[]  KbOutMin=[]  KbOutMax=[]  KtOutMin=[]  KtOutMax=[]  IntegratorOutMin=[]  IntegratorOutMax=[]  FilterOutMin=[]  FilterOutMax=[]  SumI1OutMin=[]  SumI1OutMax=[]  SumI2OutMin=[]  SumI2OutMax=[]  SumI3OutMin=[]  SumI3OutMax=[]  SumI4OutMin=[]  SumI4OutMax=[]  SumDOutMin=[]  SumDOutMax=[]  DifferentiatorOutMin=[]  DifferentiatorOutMax=[]  FilterDiffOutCoefMin=[]  FilterDiffOutCoefMax=[]  ReciprocalOutMin=[]  ReciprocalOutMax=[]  SumDenOutMin=[]  SumDenOutMax=[]  SumNumOutMin=[]  SumNumOutMax=[]  DivideOutMin=[]  DivideOutMax=[]  UdiffTsProdOutMin=[]  UdiffTsProdOutMax=[]  NTsProdOutMin=[]  NTsProdOutMax=[]  UintegralTsProdOutMin=[]  UintegralTsProdOutMax=[]  UngainTsProdOutMin=[]  UngainTsProdOutMax=[]  IntegratorContinuousStateAttributes=''  IntegratorStateMustResolveToSignalObject=off  IntegratorRTWStateStorageClass=Auto  FilterContinuousStateAttributes=''  FilterStateMustResolveToSignalObject=off  FilterRTWStateStorageClass=Auto  ParallelPVariant=InternalParameters  IdealPVariant=Disabled  IVariant=InternalParameters  DVariant=Disabled  IntegratorVariant=Continuous  SatVariant=Disabled  AWVariant=Passthrough  PCopyVariant=Disabled  TRVariant=Disabled  FdbkBlocksVariant=Forward  IdealPFdbkVariant=Disabled  SatFdbkVariant=Disabled  DerivativeFilterVariant=Disabled  NVariant=Disabled  NCopyVariant=Disabled_SignalSpec  FilterICVariant=Disabled  IntegratorICVariant=InternalICs  ExternalResetVariant=Disabled  TRSumVariant=Passthrough  SumFdbkVariant=Disabled  SumVariant=Sum_PI  TsampFilterVariant=InternalTs  TsampNgainVariant=Passthrough  TsampIntegralVariant=Passthrough  ExternalSaturationOutDataTypeStr=Inherit: Same as second input
  Product3 : Product
  Rn : powerlib/Elements/Series RLC Branch  LConnTagsString=__new0  RConnTagsString=__new0  BranchType=R  Resistance=Rn  Inductance=1e-3  SetiL0=off  InitialCurrent=0  Capacitance=1e-6  Setx0=off  InitialVoltage=0  Measurements=None
  Rn1 : powerlib/Elements/Series RLC Branch  LConnTagsString=__new0  RConnTagsString=__new0  BranchType=R  Resistance=3  Inductance=1e-3  SetiL0=off  InitialCurrent=0  Capacitance=1e-6  Setx0=off  InitialVoltage=0  Measurements=None
  Saturation : Saturate  UpperLimit=1  LowerLimit=-1
  Saturation1 : Saturate  UpperLimit=1000  LowerLimit=-1000
  Scope : Scope  NumInputPorts=4
  Scope{1..3,9} (4 alike) : Scope
  Scope4 : Scope  NumInputPorts=2
  Scope6 : Scope  NumInputPorts=2
  Sin : Trigonometry
  Sinusoidal Measurement (PLL) : eeSinusoidalMeasurementV2/Sinusoidal Measurement (PLL)  Ki_PD=1000  Kp_LF=400  Ki_LF=20000  F0=60  Theta0=0  Mag0=1  Ts=-1
      settings: SourceProductBaseCode=PS
  Subsystem1 : Subsystem
  Sum1 : Sum  Inputs=|+-
  Sum4 : Sum  Inputs=-+|
  Sum5 : Sum  Inputs=-+|
  Uref : Constant  Value=Udcref
  Voltage Measurement : powerlib/Measurements/Voltage Measurement  PhasorSimulation=off  OutputType=Complex  PSBequivalent=0
  Voltage Measurement1 : powerlib/Measurements/Voltage Measurement  PhasorSimulation=off  OutputType=Complex  PSBequivalent=0
  Un1 : PMIOPort  Side=Left
  Un2 : PMIOPort  Port=2  Side=Left
  Udc+ : PMIOPort  Port=3  Side=Right
  Udc- : PMIOPort  Port=4  Side=Right
  wires:
  Voltage Measurement1/1 -> Scope4/2, [Un]
  Current Measurement/1 -> Scope4/1, [In]
  [AN] -> IGBT/Diode1/1
  Clock/1 -> Compare To Constant/1
  Voltage Measurement/1 -> [Udc]
  Compare To Constant/1 -> IGBT/Diode4/1
  [AP] -> IGBT/Diode/1
  Current Measurement2/1 -> Scope2/1
  [BP] -> IGBT/Diode2/1
  [BN] -> IGBT/Diode3/1
  Saturation/1 -> Subsystem1/1(In1)
  Subsystem1/4(Out4) -> [BN]
  Sum1/1 -> PID Controller/1
  [In] -> Scope/4
  Subsystem1/2(Out2) -> [AN]
  [Un] -> Sinusoidal Measurement (PLL)/1
  Sum4/1 -> Gain/1, Scope9/1
  PID Controller/1 -> Saturation1/1
  [Un] -> Sum4/2
  [In] -> Sum5/1, Scope6/1
  Subsystem1/3(Out3) -> [BP]
  Product3/1 -> Sum5/2, Scope6/2
  Gain1/1 -> Scope1/1, Sum4/1
  Subsystem1/1(Out1) -> [AP]
  Gain/1 -> Saturation/1
  Sinusoidal Measurement (PLL)/2 -> Sin/1
  Uref/1 -> Sum1/1
  Sum5/1 -> Gain1/1
  [Un] -> Scope/3
  [Udc] -> Sum1/2
  Sin/1 -> Product3/1
  Saturation1/1 -> Product3/2, Scope3/1
  [Udc] -> Scope/2
  Constant/1 -> Scope/1
  connections:
  IGBT/Diode1/RConn1 -- Voltage Measurement/LConn2 -- Udc-/RConn1 -- IGBT/Diode3/RConn1
  Rn/LConn1 -- Ln/RConn1
  Current Measurement2/LConn1 -- IGBT/Diode2/LConn1 -- IGBT/Diode/LConn1
  IGBT/Diode1/LConn1 -- IGBT/Diode/RConn1 -- Current Measurement/RConn1
  IGBT/Diode4/RConn1 -- Rn1/RConn1 -- Ln/LConn1
  Rn/RConn1 -- Current Measurement/LConn1
  Voltage Measurement1/LConn1 -- Rn1/LConn1 -- IGBT/Diode4/LConn1 -- Un1/RConn1
  Voltage Measurement/LConn1 -- Udc+/RConn1 -- Current Measurement2/RConn1
  IGBT/Diode3/LConn1 -- IGBT/Diode2/RConn1 -- Un2/RConn1 -- Voltage Measurement1/LConn2

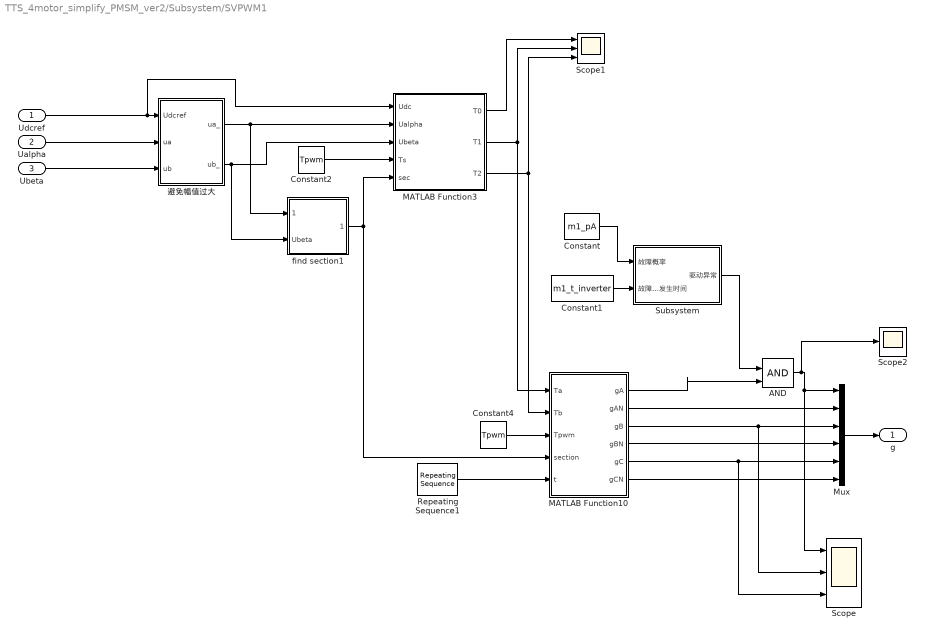
== system TTS_4motor_simplify_PMSM_ver2/Subsystem/SVPWM1 ==
  Udcref : Inport
  Ualpha : Inport  Port=2
  Ubeta : Inport  Port=3
  AND : Logic  IconShape=distinctive  AllPortsSameDT=off  OutDataTypeStr=boolean
  Constant : Constant  Value=m1_pA
  Constant1 : Constant  Value=m1_t_inverter
  Constant2 : Constant  Value=Tpwm
  Constant4 : Constant  Value=Tpwm
  MATLAB Function10 : MATLAB Function  TreatAsAtomicUnit=on
  MATLAB Function3 : MATLAB Function  TreatAsAtomicUnit=on
  Mux : Mux  Inputs=6
  Repeating Sequence1 : simulink/Sources/Repeating Sequence  rep_seq_t=[0 Tpwm]  rep_seq_y=[0 Tpwm]
  Scope : Scope  NumInputPorts=3
  Scope1 : Scope  NumInputPorts=3
  Scope2 : Scope
  Subsystem : Subsystem
  find section1 : Subsystem
  避免幅值过大 : MATLAB Function  TreatAsAtomicUnit=on
  g : Outport
  wires:
  Ualpha/1 -> 避免幅值过大/2(ua)
  Ubeta/1 -> 避免幅值过大/3(ub)
  Constant2/1 -> MATLAB Function3/4(Ts)
  MATLAB Function3/1(T0) -> Scope1/1
  Udcref/1 -> MATLAB Function3/1(Udc), 避免幅值过大/1(Udcref)
  MATLAB Function3/2(T1) -> Scope1/2, MATLAB Function10/1(Ta)
  find section1/1(section) -> MATLAB Function10/4(section), MATLAB Function3/5(sec)
  Constant4/1 -> MATLAB Function10/3(Tpwm)
  Repeating Sequence1/1 -> MATLAB Function10/5(t)
  MATLAB Function3/3(T2) -> Scope1/3, MATLAB Function10/2(Tb)
  MATLAB Function10/6(gCN) -> Mux/6
  MATLAB Function10/5(gC) -> Scope/3, Mux/5
  MATLAB Function10/4(gBN) -> Mux/4
  MATLAB Function10/3(gB) -> Scope/2, Mux/3
  MATLAB Function10/2(gAN) -> Mux/2
  Mux/1 -> g/1
  MATLAB Function10/1(gA) -> AND/2
  避免幅值过大/1(ua_) -> find section1/1(Ualpha), MATLAB Function3/2(Ualpha)
  避免幅值过大/2(ub_) -> find section1/2(Ubeta), MATLAB Function3/3(Ubeta)
  AND/1 -> Scope2/1, Scope/1, Mux/1
  Subsystem/1(驱动异常) -> AND/1
  Constant/1 -> Subsystem/1(故障概率)
  Constant1/1 -> Subsystem/2(故障发生时间)

== system TTS_4motor_simplify_PMSM_ver2/Subsystem/转速调节器ASR ==
  "  " : Inport
  Integrator Limited : Integrator  LimitOutput=on  UpperSaturationLimit=40  LowerSaturationLimit=-40
  I积分放大倍数 : Gain  Gain=0.4
  PI输出限幅1 : Saturate  UpperLimit=100  LowerLimit=-100
  P比例放大倍数 : Gain  Gain=5
  Scope : Scope  NumInputPorts=2
  Sum1 : Sum  Inputs=|++
  Te* : Outport  VectorParamsAs1DForOutWhenUnconnected=off
  wires:
  I积分放大倍数/1 -> Integrator Limited/1
  "  "/1 -> P比例放大倍数/1, I积分放大倍数/1
  Integrator Limited/1 -> Scope/2, Sum1/2
  Sum1/1 -> PI输出限幅1/1
  PI输出限幅1/1 -> Scope/1, Te*/1
  P比例放大倍数/1 -> Sum1/1

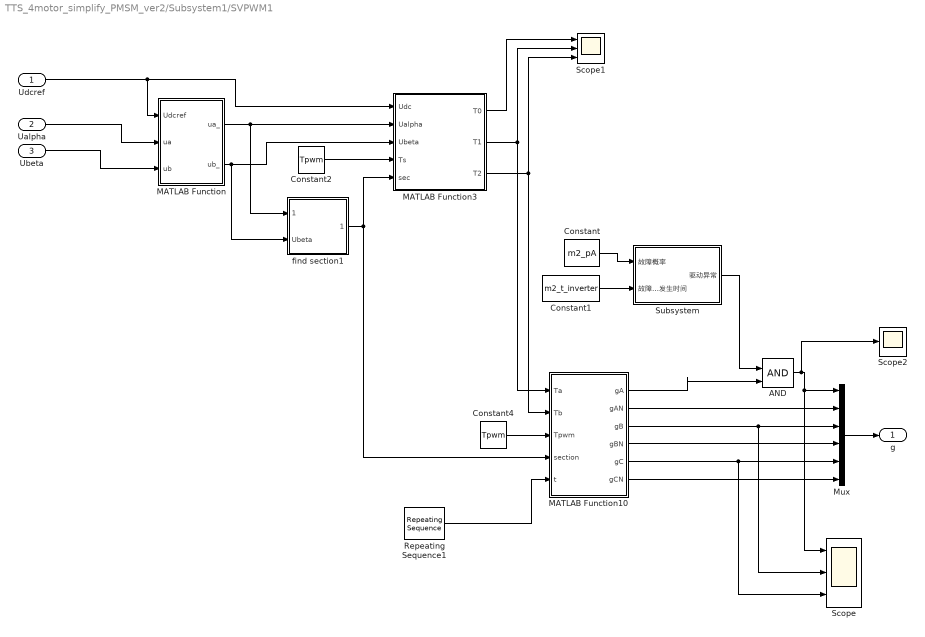
== system TTS_4motor_simplify_PMSM_ver2/Subsystem1/SVPWM1 ==
  Udcref : Inport
  Ualpha : Inport  Port=2
  Ubeta : Inport  Port=3
  AND : Logic  IconShape=distinctive  AllPortsSameDT=off  OutDataTypeStr=boolean
  Constant : Constant  Value=m2_pA
  Constant1 : Constant  Value=m2_t_inverter
  Constant2 : Constant  Value=Tpwm
  Constant4 : Constant  Value=Tpwm
  MATLAB Function : MATLAB Function  TreatAsAtomicUnit=on
  MATLAB Function10 : MATLAB Function  TreatAsAtomicUnit=on
  MATLAB Function3 : MATLAB Function  TreatAsAtomicUnit=on
  Mux : Mux  Inputs=6
  Repeating Sequence1 : simulink/Sources/Repeating Sequence  rep_seq_t=[0 Tpwm]  rep_seq_y=[0 Tpwm]
  Scope : Scope  NumInputPorts=3
  Scope1 : Scope  NumInputPorts=3
  Scope2 : Scope
  Subsystem : Subsystem
  find section1 : Subsystem
  g : Outport
  wires:
  Constant1/1 -> Subsystem/2(故障发生时间)
  Constant/1 -> Subsystem/1(故障概率)
  Subsystem/1(驱动异常) -> AND/1
  AND/1 -> Mux/1, Scope/1, Scope2/1
  MATLAB Function/2(ub_) -> MATLAB Function3/3(Ubeta), find section1/2(Ubeta)
  MATLAB Function/1(ua_) -> MATLAB Function3/2(Ualpha), find section1/1(Ualpha)
  MATLAB Function10/1(gA) -> AND/2
  Mux/1 -> g/1
  MATLAB Function10/2(gAN) -> Mux/2
  MATLAB Function10/3(gB) -> Mux/3, Scope/2
  MATLAB Function10/4(gBN) -> Mux/4
  MATLAB Function10/5(gC) -> Mux/5, Scope/3
  MATLAB Function10/6(gCN) -> Mux/6
  MATLAB Function3/3(T2) -> MATLAB Function10/2(Tb), Scope1/3
  Repeating Sequence1/1 -> MATLAB Function10/5(t)
  Constant4/1 -> MATLAB Function10/3(Tpwm)
  find section1/1(section) -> MATLAB Function3/5(sec), MATLAB Function10/4(section)
  MATLAB Function3/2(T1) -> MATLAB Function10/1(Ta), Scope1/2
  Udcref/1 -> MATLAB Function/1(Udcref), MATLAB Function3/1(Udc)
  MATLAB Function3/1(T0) -> Scope1/1
  Constant2/1 -> MATLAB Function3/4(Ts)
  Ubeta/1 -> MATLAB Function/3(ub)
  Ualpha/1 -> MATLAB Function/2(ua)

== system TTS_4motor_simplify_PMSM_ver2/Subsystem1/转速调节器ASR ==
  "  " : Inport
  Integrator Limited : Integrator  LimitOutput=on  UpperSaturationLimit=40  LowerSaturationLimit=-40
  I积分放大倍数 : Gain  Gain=0.4
  PI输出限幅1 : Saturate  UpperLimit=100  LowerLimit=-100
  P比例放大倍数 : Gain  Gain=5
  Scope : Scope  NumInputPorts=2
  Sum1 : Sum  Inputs=|++
  Te* : Outport  VectorParamsAs1DForOutWhenUnconnected=off
  wires:
  P比例放大倍数/1 -> Sum1/1
  PI输出限幅1/1 -> Te*/1, Scope/1
  Sum1/1 -> PI输出限幅1/1
  Integrator Limited/1 -> Sum1/2, Scope/2
  "  "/1 -> I积分放大倍数/1, P比例放大倍数/1
  I积分放大倍数/1 -> Integrator Limited/1

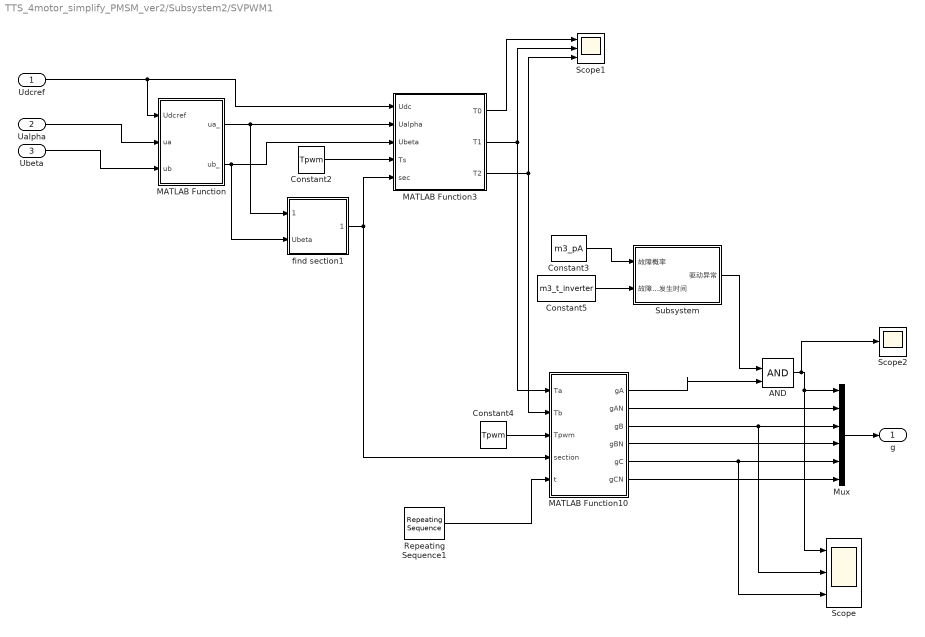
== system TTS_4motor_simplify_PMSM_ver2/Subsystem2/SVPWM1 ==
  Udcref : Inport
  Ualpha : Inport  Port=2
  Ubeta : Inport  Port=3
  AND : Logic  IconShape=distinctive  AllPortsSameDT=off  OutDataTypeStr=boolean
  Constant2 : Constant  Value=Tpwm
  Constant3 : Constant  Value=m3_pA
  Constant4 : Constant  Value=Tpwm
  Constant5 : Constant  Value=m3_t_inverter
  MATLAB Function : MATLAB Function  TreatAsAtomicUnit=on
  MATLAB Function10 : MATLAB Function  TreatAsAtomicUnit=on
  MATLAB Function3 : MATLAB Function  TreatAsAtomicUnit=on
  Mux : Mux  Inputs=6
  Repeating Sequence1 : simulink/Sources/Repeating Sequence  rep_seq_t=[0 Tpwm]  rep_seq_y=[0 Tpwm]
  Scope : Scope  NumInputPorts=3
  Scope1 : Scope  NumInputPorts=3
  Scope2 : Scope
  Subsystem : Subsystem
  find section1 : Subsystem
  g : Outport
  wires:
  Ualpha/1 -> MATLAB Function/2(ua)
  Ubeta/1 -> MATLAB Function/3(ub)
  Constant2/1 -> MATLAB Function3/4(Ts)
  MATLAB Function3/1(T0) -> Scope1/1
  Udcref/1 -> MATLAB Function3/1(Udc), MATLAB Function/1(Udcref)
  MATLAB Function3/2(T1) -> Scope1/2, MATLAB Function10/1(Ta)
  find section1/1(section) -> MATLAB Function10/4(section), MATLAB Function3/5(sec)
  Constant4/1 -> MATLAB Function10/3(Tpwm)
  Repeating Sequence1/1 -> MATLAB Function10/5(t)
  MATLAB Function3/3(T2) -> Scope1/3, MATLAB Function10/2(Tb)
  MATLAB Function10/6(gCN) -> Mux/6
  MATLAB Function10/5(gC) -> Scope/3, Mux/5
  MATLAB Function10/4(gBN) -> Mux/4
  MATLAB Function10/3(gB) -> Scope/2, Mux/3
  MATLAB Function10/2(gAN) -> Mux/2
  Mux/1 -> g/1
  MATLAB Function10/1(gA) -> AND/2
  MATLAB Function/1(ua_) -> find section1/1(Ualpha), MATLAB Function3/2(Ualpha)
  MATLAB Function/2(ub_) -> find section1/2(Ubeta), MATLAB Function3/3(Ubeta)
  AND/1 -> Scope2/1, Scope/1, Mux/1
  Subsystem/1(驱动异常) -> AND/1
  Constant5/1 -> Subsystem/2(故障发生时间)
  Constant3/1 -> Subsystem/1(故障概率)

== system TTS_4motor_simplify_PMSM_ver2/Subsystem2/转速调节器ASR ==
  "  " : Inport
  Integrator Limited : Integrator  LimitOutput=on  UpperSaturationLimit=40  LowerSaturationLimit=-40
  I积分放大倍数 : Gain  Gain=0.4
  PI输出限幅1 : Saturate  UpperLimit=100  LowerLimit=-100
  P比例放大倍数 : Gain  Gain=5
  Scope : Scope  NumInputPorts=2
  Sum1 : Sum  Inputs=|++
  Te* : Outport  VectorParamsAs1DForOutWhenUnconnected=off
  wires:
  I积分放大倍数/1 -> Integrator Limited/1
  "  "/1 -> P比例放大倍数/1, I积分放大倍数/1
  Integrator Limited/1 -> Scope/2, Sum1/2
  Sum1/1 -> PI输出限幅1/1
  PI输出限幅1/1 -> Scope/1, Te*/1
  P比例放大倍数/1 -> Sum1/1

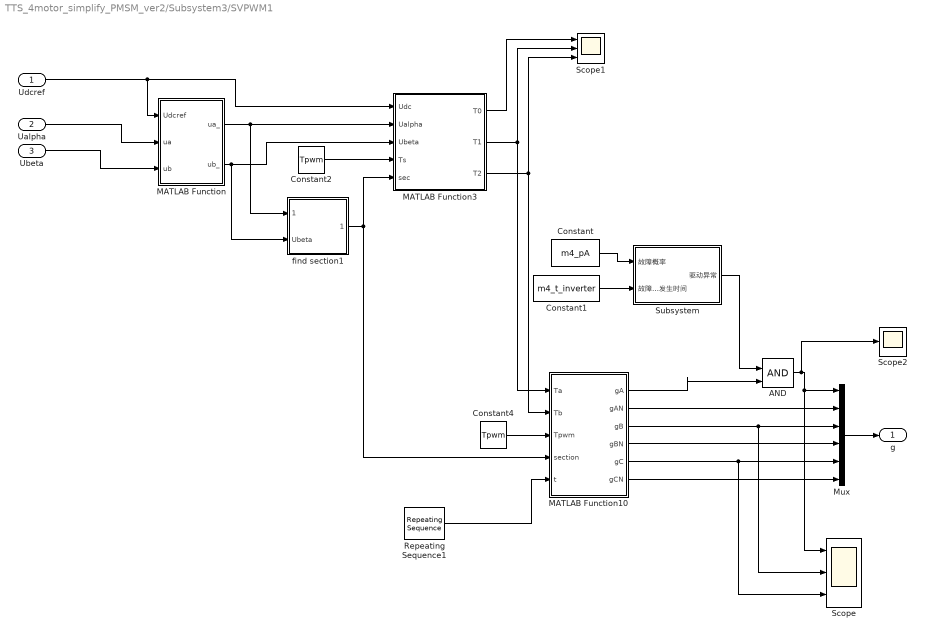
== system TTS_4motor_simplify_PMSM_ver2/Subsystem3/SVPWM1 ==
  Udcref : Inport
  Ualpha : Inport  Port=2
  Ubeta : Inport  Port=3
  AND : Logic  IconShape=distinctive  AllPortsSameDT=off  OutDataTypeStr=boolean
  Constant : Constant  Value=m4_pA
  Constant1 : Constant  Value=m4_t_inverter
  Constant2 : Constant  Value=Tpwm
  Constant4 : Constant  Value=Tpwm
  MATLAB Function : MATLAB Function  TreatAsAtomicUnit=on
  MATLAB Function10 : MATLAB Function  TreatAsAtomicUnit=on
  MATLAB Function3 : MATLAB Function  TreatAsAtomicUnit=on
  Mux : Mux  Inputs=6
  Repeating Sequence1 : simulink/Sources/Repeating Sequence  rep_seq_t=[0 Tpwm]  rep_seq_y=[0 Tpwm]
  Scope : Scope  NumInputPorts=3
  Scope1 : Scope  NumInputPorts=3
  Scope2 : Scope
  Subsystem : Subsystem
  find section1 : Subsystem
  g : Outport
  wires:
  Constant1/1 -> Subsystem/2(故障发生时间)
  Constant/1 -> Subsystem/1(故障概率)
  Subsystem/1(驱动异常) -> AND/1
  AND/1 -> Mux/1, Scope/1, Scope2/1
  MATLAB Function/2(ub_) -> MATLAB Function3/3(Ubeta), find section1/2(Ubeta)
  MATLAB Function/1(ua_) -> MATLAB Function3/2(Ualpha), find section1/1(Ualpha)
  MATLAB Function10/1(gA) -> AND/2
  Mux/1 -> g/1
  MATLAB Function10/2(gAN) -> Mux/2
  MATLAB Function10/3(gB) -> Mux/3, Scope/2
  MATLAB Function10/4(gBN) -> Mux/4
  MATLAB Function10/5(gC) -> Mux/5, Scope/3
  MATLAB Function10/6(gCN) -> Mux/6
  MATLAB Function3/3(T2) -> MATLAB Function10/2(Tb), Scope1/3
  Repeating Sequence1/1 -> MATLAB Function10/5(t)
  Constant4/1 -> MATLAB Function10/3(Tpwm)
  find section1/1(section) -> MATLAB Function3/5(sec), MATLAB Function10/4(section)
  MATLAB Function3/2(T1) -> MATLAB Function10/1(Ta), Scope1/2
  Udcref/1 -> MATLAB Function/1(Udcref), MATLAB Function3/1(Udc)
  MATLAB Function3/1(T0) -> Scope1/1
  Constant2/1 -> MATLAB Function3/4(Ts)
  Ubeta/1 -> MATLAB Function/3(ub)
  Ualpha/1 -> MATLAB Function/2(ua)

== system TTS_4motor_simplify_PMSM_ver2/Subsystem3/转速调节器ASR ==
  "  " : Inport
  Integrator Limited : Integrator  LimitOutput=on  UpperSaturationLimit=40  LowerSaturationLimit=-40
  I积分放大倍数 : Gain  Gain=0.4
  PI输出限幅1 : Saturate  UpperLimit=100  LowerLimit=-100
  P比例放大倍数 : Gain  Gain=5
  Scope : Scope  NumInputPorts=2
  Sum1 : Sum  Inputs=|++
  Te* : Outport  VectorParamsAs1DForOutWhenUnconnected=off
  wires:
  P比例放大倍数/1 -> Sum1/1
  PI输出限幅1/1 -> Te*/1, Scope/1
  Sum1/1 -> PI输出限幅1/1
  Integrator Limited/1 -> Sum1/2, Scope/2
  "  "/1 -> I积分放大倍数/1, P比例放大倍数/1
  I积分放大倍数/1 -> Integrator Limited/1

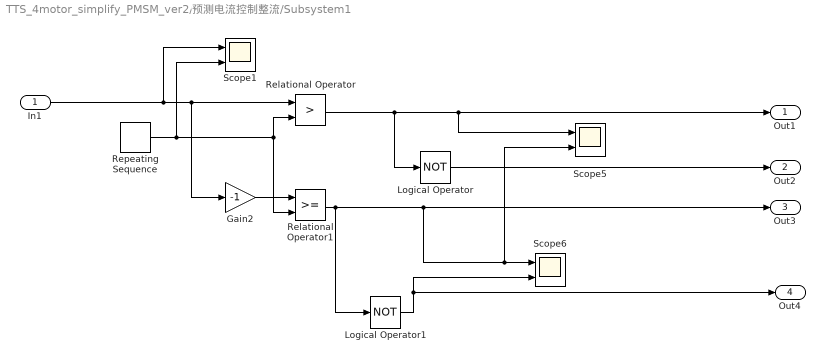
== system TTS_4motor_simplify_PMSM_ver2/预测电流控制整流/Subsystem1 ==
  In1 : Inport
  Gain2 : Gain  Gain=-1
  Logical Operator : Logic  Operator=NOT  AllPortsSameDT=off  OutDataTypeStr=boolean
  Logical Operator1 : Logic  Operator=NOT  AllPortsSameDT=off  OutDataTypeStr=boolean
  Relational Operator : RelationalOperator  Operator=>  OutDataTypeStr=boolean  RndMeth=Simplest
  Relational Operator1 : RelationalOperator  OutDataTypeStr=boolean  RndMeth=Simplest
  Repeating Sequence : simulink/Sources/Repeating Sequence  rep_seq_t=[0 Tpwm/2 Tpwm]  rep_seq_y=[-1 1 -1]
  Scope1 : Scope  NumInputPorts=2
  Scope5 : Scope  NumInputPorts=2
  Scope6 : Scope  NumInputPorts=2
  Out1 : Outport
  Out2 : Outport  Port=2
  Out3 : Outport  Port=3
  Out4 : Outport  Port=4
  wires:
  Relational Operator1/1 -> Logical Operator1/1, Out3/1, Scope5/2, Scope6/1
  Gain2/1 -> Relational Operator1/1
  Relational Operator/1 -> Logical Operator/1, Out1/1, Scope5/1
  In1/1 -> Scope1/1, Gain2/1, Relational Operator/1
  Logical Operator1/1 -> Out4/1, Scope6/2
  Repeating Sequence/1 -> Scope1/2, Relational Operator1/2, Relational Operator/2
  Logical Operator/1 -> Out2/1

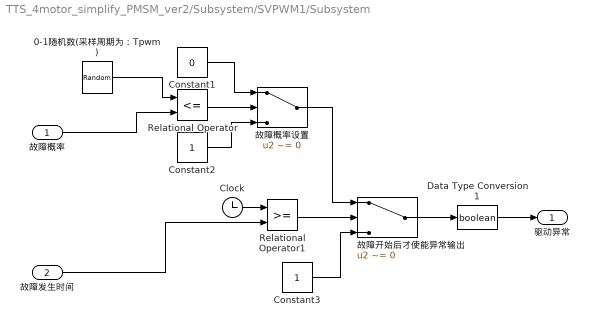
== system TTS_4motor_simplify_PMSM_ver2/Subsystem/SVPWM1/Subsystem ==
  故障概率 : Inport
  故障发生时间 : Inport  Port=2
  0-1随机数(采样周期为：Tpwm) : UniformRandomNumber  Minimum=0  SampleTime=Tpwm
  Clock : Clock
  Constant1 : Constant  Value=0
  Constant2 : Constant
  Constant3 : Constant
  Data Type Conversion1 : DataTypeConversion  OutDataTypeStr=boolean
  Relational Operator : RelationalOperator  Operator=<=  OutDataTypeStr=boolean  RndMeth=Simplest
  Relational Operator1 : RelationalOperator  OutDataTypeStr=boolean  RndMeth=Simplest
  故障开始后才使能异常输出 : Switch  Criteria=u2 ~= 0  Threshold=0.45
  故障概率设置 : Switch  Criteria=u2 ~= 0  Threshold=0.1
  驱动异常 : Outport
  wires:
  Constant3/1 -> 故障开始后才使能异常输出/3
  故障概率设置/1 -> 故障开始后才使能异常输出/1
  故障开始后才使能异常输出/1 -> Data Type Conversion1/1
  Constant1/1 -> 故障概率设置/1
  Constant2/1 -> 故障概率设置/3
  Data Type Conversion1/1 -> 驱动异常/1
  Clock/1 -> Relational Operator1/1
  Relational Operator/1 -> 故障概率设置/2
  0-1随机数(采样周期为：Tpwm)/1 -> Relational Operator/1
  故障概率/1 -> Relational Operator/2
  故障发生时间/1 -> Relational Operator1/2
  Relational Operator1/1 -> 故障开始后才使能异常输出/2

== system TTS_4motor_simplify_PMSM_ver2/Subsystem/SVPWM1/find section1 ==
  Ualpha : Inport
  Ubeta : Inport  Port=2
  >=0? : Subsystem
  Gain : Gain  Gain=sqrt(3)
  Gain1 : Gain  Gain=4
  Gain2 : Gain  Gain=2
  Sum : Sum  Inputs=++|
  Sum1 : Sum  Inputs=-+|
  Sum2 : Sum  Inputs=+++
  get section : MATLAB Function  TreatAsAtomicUnit=on
  not neg : Subsystem
  not neg1 : Subsystem
  section : Outport
  wires:
  Gain2/1 -> Sum2/2
  get section/1(y) -> section/1
  Ubeta/1 -> >=0?/1(In1), Sum1/2, Sum/2
  Gain/1 -> Sum1/1, Sum/1
  Gain1/1 -> Sum2/3
  Sum1/1 -> not neg/1(In1)
  Sum/1 -> not neg1/1(In1)
  >=0?/1(Out1) -> Gain1/1
  not neg1/1(Out1) -> Sum2/1
  Sum2/1 -> get section/1(u)
  not neg/1(Out1) -> Gain2/1
  Ualpha/1 -> Gain/1

== system TTS_4motor_simplify_PMSM_ver2/Subsystem1/SVPWM1/Subsystem ==
  故障概率 : Inport
  故障发生时间 : Inport  Port=2
  0-1随机数(采样周期为：Tpwm) : UniformRandomNumber  Minimum=0  Maximum=2  SampleTime=Tpwm
  Clock : Clock
  Constant1 : Constant  Value=0
  Constant2 : Constant
  Constant3 : Constant
  Data Type Conversion1 : DataTypeConversion  OutDataTypeStr=boolean
  Relational Operator : RelationalOperator  Operator=<=  OutDataTypeStr=boolean  RndMeth=Simplest
  Relational Operator1 : RelationalOperator  OutDataTypeStr=boolean  RndMeth=Simplest
  故障开始后才使能异常输出 : Switch  Criteria=u2 ~= 0  Threshold=0.45
  故障概率设置 : Switch  Criteria=u2 ~= 0  Threshold=0.1
  驱动异常 : Outport
  wires:
  Relational Operator1/1 -> 故障开始后才使能异常输出/2
  故障发生时间/1 -> Relational Operator1/2
  故障概率/1 -> Relational Operator/2
  0-1随机数(采样周期为：Tpwm)/1 -> Relational Operator/1
  Relational Operator/1 -> 故障概率设置/2
  Clock/1 -> Relational Operator1/1
  Data Type Conversion1/1 -> 驱动异常/1
  Constant2/1 -> 故障概率设置/3
  Constant1/1 -> 故障概率设置/1
  故障开始后才使能异常输出/1 -> Data Type Conversion1/1
  故障概率设置/1 -> 故障开始后才使能异常输出/1
  Constant3/1 -> 故障开始后才使能异常输出/3

== system TTS_4motor_simplify_PMSM_ver2/Subsystem1/SVPWM1/find section1 ==
  Ualpha : Inport
  Ubeta : Inport  Port=2
  >=0? : Subsystem
  Gain : Gain  Gain=sqrt(3)
  Gain1 : Gain  Gain=4
  Gain2 : Gain  Gain=2
  Sum : Sum  Inputs=++|
  Sum1 : Sum  Inputs=-+|
  Sum2 : Sum  Inputs=+++
  get section : MATLAB Function  TreatAsAtomicUnit=on
  not neg : Subsystem
  not neg1 : Subsystem
  section : Outport
  wires:
  Ualpha/1 -> Gain/1
  not neg/1(Out1) -> Gain2/1
  Sum2/1 -> get section/1(u)
  not neg1/1(Out1) -> Sum2/1
  >=0?/1(Out1) -> Gain1/1
  Sum/1 -> not neg1/1(In1)
  Sum1/1 -> not neg/1(In1)
  Gain1/1 -> Sum2/3
  Gain/1 -> Sum/1, Sum1/1
  Ubeta/1 -> Sum/2, Sum1/2, >=0?/1(In1)
  get section/1(y) -> section/1
  Gain2/1 -> Sum2/2

== system TTS_4motor_simplify_PMSM_ver2/Subsystem2/SVPWM1/Subsystem ==
  故障概率 : Inport
  故障发生时间 : Inport  Port=2
  0-1随机数(采样周期为：Tpwm) : UniformRandomNumber  Minimum=0  Seed=3  SampleTime=Tpwm
  Clock : Clock
  Constant1 : Constant  Value=0
  Constant2 : Constant
  Constant3 : Constant
  Data Type Conversion1 : DataTypeConversion  OutDataTypeStr=boolean
  Relational Operator : RelationalOperator  Operator=<=  OutDataTypeStr=boolean  RndMeth=Simplest
  Relational Operator1 : RelationalOperator  OutDataTypeStr=boolean  RndMeth=Simplest
  故障开始后才使能异常输出 : Switch  Criteria=u2 ~= 0  Threshold=0.45
  故障概率设置 : Switch  Criteria=u2 ~= 0  Threshold=0.1
  驱动异常 : Outport
  wires:
  Constant3/1 -> 故障开始后才使能异常输出/3
  故障概率设置/1 -> 故障开始后才使能异常输出/1
  故障开始后才使能异常输出/1 -> Data Type Conversion1/1
  Constant1/1 -> 故障概率设置/1
  Constant2/1 -> 故障概率设置/3
  Data Type Conversion1/1 -> 驱动异常/1
  Clock/1 -> Relational Operator1/1
  Relational Operator/1 -> 故障概率设置/2
  0-1随机数(采样周期为：Tpwm)/1 -> Relational Operator/1
  故障概率/1 -> Relational Operator/2
  故障发生时间/1 -> Relational Operator1/2
  Relational Operator1/1 -> 故障开始后才使能异常输出/2

== system TTS_4motor_simplify_PMSM_ver2/Subsystem2/SVPWM1/find section1 ==
  Ualpha : Inport
  Ubeta : Inport  Port=2
  >=0? : Subsystem
  Gain : Gain  Gain=sqrt(3)
  Gain1 : Gain  Gain=4
  Gain2 : Gain  Gain=2
  Sum : Sum  Inputs=++|
  Sum1 : Sum  Inputs=-+|
  Sum2 : Sum  Inputs=+++
  get section : MATLAB Function  TreatAsAtomicUnit=on
  not neg : Subsystem
  not neg1 : Subsystem
  section : Outport
  wires:
  Gain2/1 -> Sum2/2
  get section/1(y) -> section/1
  Ubeta/1 -> >=0?/1(In1), Sum1/2, Sum/2
  Gain/1 -> Sum1/1, Sum/1
  Gain1/1 -> Sum2/3
  Sum1/1 -> not neg/1(In1)
  Sum/1 -> not neg1/1(In1)
  >=0?/1(Out1) -> Gain1/1
  not neg1/1(Out1) -> Sum2/1
  Sum2/1 -> get section/1(u)
  not neg/1(Out1) -> Gain2/1
  Ualpha/1 -> Gain/1

== system TTS_4motor_simplify_PMSM_ver2/Subsystem3/SVPWM1/Subsystem ==
  故障概率 : Inport
  故障发生时间 : Inport  Port=2
  0-1随机数(采样周期为：Tpwm) : UniformRandomNumber  Minimum=0  Seed=4  SampleTime=Tpwm
  Clock : Clock
  Constant1 : Constant  Value=0
  Constant2 : Constant
  Constant3 : Constant
  Data Type Conversion1 : DataTypeConversion  OutDataTypeStr=boolean
  Relational Operator : RelationalOperator  Operator=<=  OutDataTypeStr=boolean  RndMeth=Simplest
  Relational Operator1 : RelationalOperator  OutDataTypeStr=boolean  RndMeth=Simplest
  故障开始后才使能异常输出 : Switch  Criteria=u2 ~= 0  Threshold=0.45
  故障概率设置 : Switch  Criteria=u2 ~= 0  Threshold=0.1
  驱动异常 : Outport
  wires:
  Relational Operator1/1 -> 故障开始后才使能异常输出/2
  故障发生时间/1 -> Relational Operator1/2
  故障概率/1 -> Relational Operator/2
  0-1随机数(采样周期为：Tpwm)/1 -> Relational Operator/1
  Relational Operator/1 -> 故障概率设置/2
  Clock/1 -> Relational Operator1/1
  Data Type Conversion1/1 -> 驱动异常/1
  Constant2/1 -> 故障概率设置/3
  Constant1/1 -> 故障概率设置/1
  故障开始后才使能异常输出/1 -> Data Type Conversion1/1
  故障概率设置/1 -> 故障开始后才使能异常输出/1
  Constant3/1 -> 故障开始后才使能异常输出/3

== system TTS_4motor_simplify_PMSM_ver2/Subsystem3/SVPWM1/find section1 ==
  Ualpha : Inport
  Ubeta : Inport  Port=2
  >=0? : Subsystem
  Gain : Gain  Gain=sqrt(3)
  Gain1 : Gain  Gain=4
  Gain2 : Gain  Gain=2
  Sum : Sum  Inputs=++|
  Sum1 : Sum  Inputs=-+|
  Sum2 : Sum  Inputs=+++
  get section : MATLAB Function  TreatAsAtomicUnit=on
  not neg : Subsystem
  not neg1 : Subsystem
  section : Outport
  wires:
  Ualpha/1 -> Gain/1
  not neg/1(Out1) -> Gain2/1
  Sum2/1 -> get section/1(u)
  not neg1/1(Out1) -> Sum2/1
  >=0?/1(Out1) -> Gain1/1
  Sum/1 -> not neg1/1(In1)
  Sum1/1 -> not neg/1(In1)
  Gain1/1 -> Sum2/3
  Gain/1 -> Sum/1, Sum1/1
  Ubeta/1 -> Sum/2, Sum1/2, >=0?/1(In1)
  get section/1(y) -> section/1
  Gain2/1 -> Sum2/2

== system TTS_4motor_simplify_PMSM_ver2/Subsystem/SVPWM1/find section1/>=0? ==
  In1 : Inport
  Constant2 : Constant  Value=0
  Relational Operator : RelationalOperator  OutDataTypeStr=boolean  RndMeth=Simplest
  Out1 : Outport
  wires:
  Constant2/1 -> Relational Operator/2
  Relational Operator/1 -> Out1/1
  In1/1 -> Relational Operator/1
